simulink model "PONG"  (R2018b)
settings: Solver=VariableStepAuto  StartTime=0.0  StopTime=10  RelTol=1e-3
libraries: simulink_extras x28
(part 2 of 3)

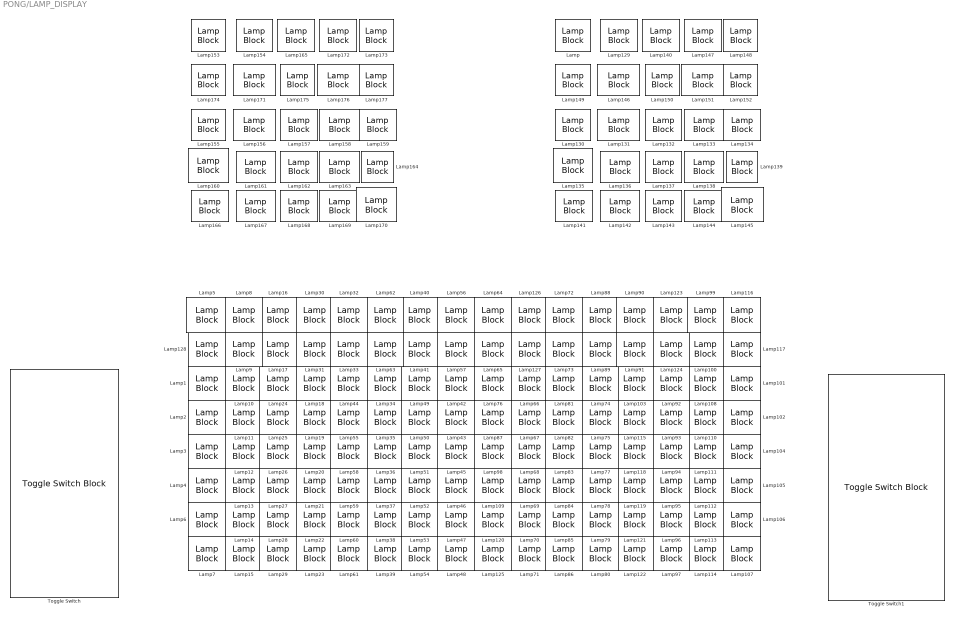
== system PONG/LAMP_DISPLAY  ==
  Lamp : LampBlock  WebBlockId=4723  LabelPosition=Hide
  Lamp1 : LampBlock  WebBlockId=1763  LabelPosition=Hide
  Lamp10 : LampBlock  WebBlockId=1211  LabelPosition=Hide
  Lamp100 : LampBlock  WebBlockId=1301  LabelPosition=Hide
  Lamp101 : LampBlock  WebBlockId=1302  LabelPosition=Hide
  Lamp102 : LampBlock  WebBlockId=1303  LabelPosition=Hide
  Lamp103 : LampBlock  WebBlockId=1304  LabelPosition=Hide
  Lamp104 : LampBlock  WebBlockId=1305  LabelPosition=Hide
  Lamp105 : LampBlock  WebBlockId=1306  LabelPosition=Hide
  Lamp106 : LampBlock  WebBlockId=1307  LabelPosition=Hide
  Lamp107 : LampBlock  WebBlockId=1308  LabelPosition=Hide
  Lamp108 : LampBlock  WebBlockId=1309  LabelPosition=Hide
  Lamp109 : LampBlock  WebBlockId=1310  LabelPosition=Hide
  Lamp11 : LampBlock  WebBlockId=1212  LabelPosition=Hide
  Lamp110 : LampBlock  WebBlockId=1311  LabelPosition=Hide
  Lamp111 : LampBlock  WebBlockId=1312  LabelPosition=Hide
  Lamp112 : LampBlock  WebBlockId=1313  LabelPosition=Hide
  Lamp113 : LampBlock  WebBlockId=1314  LabelPosition=Hide
  Lamp114 : LampBlock  WebBlockId=1315  LabelPosition=Hide
  Lamp115 : LampBlock  WebBlockId=1316  LabelPosition=Hide
  Lamp116 : LampBlock  WebBlockId=1317  LabelPosition=Hide
  Lamp117 : LampBlock  WebBlockId=1318  LabelPosition=Hide
  Lamp118 : LampBlock  WebBlockId=1319  LabelPosition=Hide
  Lamp119 : LampBlock  WebBlockId=1320  LabelPosition=Hide
  Lamp12 : LampBlock  WebBlockId=1213  LabelPosition=Hide
  Lamp120 : LampBlock  WebBlockId=1321  LabelPosition=Hide
  Lamp121 : LampBlock  WebBlockId=1322  LabelPosition=Hide
  Lamp122 : LampBlock  WebBlockId=1323  LabelPosition=Hide
  Lamp123 : LampBlock  WebBlockId=1324  LabelPosition=Hide
  Lamp124 : LampBlock  WebBlockId=1325  LabelPosition=Hide
  Lamp125 : LampBlock  WebBlockId=1326  LabelPosition=Hide
  Lamp126 : LampBlock  WebBlockId=1327  LabelPosition=Hide
  Lamp127 : LampBlock  WebBlockId=1328  LabelPosition=Hide
  Lamp128 : LampBlock  WebBlockId=1768  LabelPosition=Hide
  Lamp129 : LampBlock  WebBlockId=4724  LabelPosition=Hide
  Lamp13 : LampBlock  WebBlockId=1214  LabelPosition=Hide
  Lamp130 : LampBlock  WebBlockId=4725  LabelPosition=Hide
  Lamp131 : LampBlock  WebBlockId=4726  LabelPosition=Hide
  Lamp132 : LampBlock  WebBlockId=4727  LabelPosition=Hide
  Lamp133 : LampBlock  WebBlockId=4728  LabelPosition=Hide
  Lamp134 : LampBlock  WebBlockId=4729  LabelPosition=Hide
  Lamp135 : LampBlock  WebBlockId=4730  LabelPosition=Hide
  Lamp136 : LampBlock  WebBlockId=4731  LabelPosition=Hide
  Lamp137 : LampBlock  WebBlockId=4732  LabelPosition=Hide
  Lamp138 : LampBlock  WebBlockId=4733  LabelPosition=Hide
  Lamp139 : LampBlock  WebBlockId=4734  LabelPosition=Hide
  Lamp14 : LampBlock  WebBlockId=1215  LabelPosition=Hide
  Lamp140 : LampBlock  WebBlockId=4735  LabelPosition=Hide
  Lamp141 : LampBlock  WebBlockId=4736  LabelPosition=Hide
  Lamp142 : LampBlock  WebBlockId=4737  LabelPosition=Hide
  Lamp143 : LampBlock  WebBlockId=4738  LabelPosition=Hide
  Lamp144 : LampBlock  WebBlockId=4739  LabelPosition=Hide
  Lamp145 : LampBlock  WebBlockId=4740  LabelPosition=Hide
  Lamp146 : LampBlock  WebBlockId=4741  LabelPosition=Hide
  Lamp147 : LampBlock  WebBlockId=4742  LabelPosition=Hide
  Lamp148 : LampBlock  WebBlockId=4743  LabelPosition=Hide
  Lamp149 : LampBlock  WebBlockId=4744  LabelPosition=Hide
  Lamp15 : LampBlock  WebBlockId=1216  LabelPosition=Hide
  Lamp150 : LampBlock  WebBlockId=4745  LabelPosition=Hide
  Lamp151 : LampBlock  WebBlockId=4746  LabelPosition=Hide
  Lamp152 : LampBlock  WebBlockId=4747  LabelPosition=Hide
  Lamp153 : LampBlock  WebBlockId=4748  LabelPosition=Hide
  Lamp154 : LampBlock  WebBlockId=4749  LabelPosition=Hide
  Lamp155 : LampBlock  WebBlockId=4750  LabelPosition=Hide
  Lamp156 : LampBlock  WebBlockId=4751  LabelPosition=Hide
  Lamp157 : LampBlock  WebBlockId=4752  LabelPosition=Hide
  Lamp158 : LampBlock  WebBlockId=4753  LabelPosition=Hide
  Lamp159 : LampBlock  WebBlockId=4754  LabelPosition=Hide
  Lamp16 : LampBlock  WebBlockId=1217  LabelPosition=Hide
  Lamp160 : LampBlock  WebBlockId=4755  LabelPosition=Hide
  Lamp161 : LampBlock  WebBlockId=4756  LabelPosition=Hide
  Lamp162 : LampBlock  WebBlockId=4757  LabelPosition=Hide
  Lamp163 : LampBlock  WebBlockId=4758  LabelPosition=Hide
  Lamp164 : LampBlock  WebBlockId=4759  LabelPosition=Hide
  Lamp165 : LampBlock  WebBlockId=4760  LabelPosition=Hide
  Lamp166 : LampBlock  WebBlockId=4761  LabelPosition=Hide
  Lamp167 : LampBlock  WebBlockId=4762  LabelPosition=Hide
  Lamp168 : LampBlock  WebBlockId=4763  LabelPosition=Hide
  Lamp169 : LampBlock  WebBlockId=4764  LabelPosition=Hide
  Lamp17 : LampBlock  WebBlockId=1218  LabelPosition=Hide
  Lamp170 : LampBlock  WebBlockId=4765  LabelPosition=Hide
  Lamp171 : LampBlock  WebBlockId=4766  LabelPosition=Hide
  Lamp172 : LampBlock  WebBlockId=4767  LabelPosition=Hide
  Lamp173 : LampBlock  WebBlockId=4768  LabelPosition=Hide
  Lamp174 : LampBlock  WebBlockId=4769  LabelPosition=Hide
  Lamp175 : LampBlock  WebBlockId=4770  LabelPosition=Hide
  Lamp176 : LampBlock  WebBlockId=4771  LabelPosition=Hide
  Lamp177 : LampBlock  WebBlockId=4772  LabelPosition=Hide
  Lamp18 : LampBlock  WebBlockId=1219  LabelPosition=Hide
  Lamp19 : LampBlock  WebBlockId=1220  LabelPosition=Hide
  Lamp2 : LampBlock  WebBlockId=1764  LabelPosition=Hide
  Lamp20 : LampBlock  WebBlockId=1221  LabelPosition=Hide
  Lamp21 : LampBlock  WebBlockId=1222  LabelPosition=Hide
  Lamp22 : LampBlock  WebBlockId=1223  LabelPosition=Hide
  Lamp23 : LampBlock  WebBlockId=1224  LabelPosition=Hide
  Lamp24 : LampBlock  WebBlockId=1225  LabelPosition=Hide
  Lamp25 : LampBlock  WebBlockId=1226  LabelPosition=Hide
  Lamp26 : LampBlock  WebBlockId=1227  LabelPosition=Hide
  Lamp27 : LampBlock  WebBlockId=1228  LabelPosition=Hide
  Lamp28 : LampBlock  WebBlockId=1229  LabelPosition=Hide
  Lamp29 : LampBlock  WebBlockId=1230  LabelPosition=Hide
  Lamp3 : LampBlock  WebBlockId=1765  LabelPosition=Hide
  Lamp30 : LampBlock  WebBlockId=1231  LabelPosition=Hide
  Lamp31 : LampBlock  WebBlockId=1232  LabelPosition=Hide
  Lamp32 : LampBlock  WebBlockId=1233  LabelPosition=Hide
  Lamp33 : LampBlock  WebBlockId=1234  LabelPosition=Hide
  Lamp34 : LampBlock  WebBlockId=1235  LabelPosition=Hide
  Lamp35 : LampBlock  WebBlockId=1236  LabelPosition=Hide
  Lamp36 : LampBlock  WebBlockId=1237  LabelPosition=Hide
  Lamp37 : LampBlock  WebBlockId=1238  LabelPosition=Hide
  Lamp38 : LampBlock  WebBlockId=1239  LabelPosition=Hide
  Lamp39 : LampBlock  WebBlockId=1240  LabelPosition=Hide
  Lamp4 : LampBlock  WebBlockId=1766  LabelPosition=Hide
  Lamp40 : LampBlock  WebBlockId=1241  LabelPosition=Hide
  Lamp41 : LampBlock  WebBlockId=1242  LabelPosition=Hide
  Lamp42 : LampBlock  WebBlockId=1243  LabelPosition=Hide
  Lamp43 : LampBlock  WebBlockId=1244  LabelPosition=Hide
  Lamp44 : LampBlock  WebBlockId=1245  LabelPosition=Hide
  Lamp45 : LampBlock  WebBlockId=1246  LabelPosition=Hide
  Lamp46 : LampBlock  WebBlockId=1247  LabelPosition=Hide
  Lamp47 : LampBlock  WebBlockId=1248  LabelPosition=Hide
  Lamp48 : LampBlock  WebBlockId=1249  LabelPosition=Hide
  Lamp49 : LampBlock  WebBlockId=1250  LabelPosition=Hide
  Lamp5 : LampBlock  WebBlockId=1767  LabelPosition=Hide
  Lamp50 : LampBlock  WebBlockId=1251  LabelPosition=Hide
  Lamp51 : LampBlock  WebBlockId=1252  LabelPosition=Hide
  Lamp52 : LampBlock  WebBlockId=1253  LabelPosition=Hide
  Lamp53 : LampBlock  WebBlockId=1254  LabelPosition=Hide
  Lamp54 : LampBlock  WebBlockId=1255  LabelPosition=Hide
  Lamp55 : LampBlock  WebBlockId=1256  LabelPosition=Hide
  Lamp56 : LampBlock  WebBlockId=1257  LabelPosition=Hide
  Lamp57 : LampBlock  WebBlockId=1258  LabelPosition=Hide
  Lamp58 : LampBlock  WebBlockId=1259  LabelPosition=Hide
  Lamp59 : LampBlock  WebBlockId=1260  LabelPosition=Hide
  Lamp6 : LampBlock  WebBlockId=1207  LabelPosition=Hide
  Lamp60 : LampBlock  WebBlockId=1261  LabelPosition=Hide
  Lamp61 : LampBlock  WebBlockId=1262  LabelPosition=Hide
  Lamp62 : LampBlock  WebBlockId=1263  LabelPosition=Hide
  Lamp63 : LampBlock  WebBlockId=1264  LabelPosition=Hide
  Lamp64 : LampBlock  WebBlockId=1265  LabelPosition=Hide
  Lamp65 : LampBlock  WebBlockId=1266  LabelPosition=Hide
  Lamp66 : LampBlock  WebBlockId=1267  LabelPosition=Hide
  Lamp67 : LampBlock  WebBlockId=1268  LabelPosition=Hide
  Lamp68 : LampBlock  WebBlockId=1269  LabelPosition=Hide
  Lamp69 : LampBlock  WebBlockId=1270  LabelPosition=Hide
  Lamp7 : LampBlock  WebBlockId=1208  LabelPosition=Hide
  Lamp70 : LampBlock  WebBlockId=1271  LabelPosition=Hide
  Lamp71 : LampBlock  WebBlockId=1272  LabelPosition=Hide
  Lamp72 : LampBlock  WebBlockId=1273  LabelPosition=Hide
  Lamp73 : LampBlock  WebBlockId=1274  LabelPosition=Hide
  Lamp74 : LampBlock  WebBlockId=1275  LabelPosition=Hide
  Lamp75 : LampBlock  WebBlockId=1276  LabelPosition=Hide
  Lamp76 : LampBlock  WebBlockId=1277  LabelPosition=Hide
  Lamp77 : LampBlock  WebBlockId=1278  LabelPosition=Hide
  Lamp78 : LampBlock  WebBlockId=1279  LabelPosition=Hide
  Lamp79 : LampBlock  WebBlockId=1280  LabelPosition=Hide
  Lamp8 : LampBlock  WebBlockId=1209  LabelPosition=Hide
  Lamp80 : LampBlock  WebBlockId=1281  LabelPosition=Hide
  Lamp81 : LampBlock  WebBlockId=1282  LabelPosition=Hide
  Lamp82 : LampBlock  WebBlockId=1283  LabelPosition=Hide
  Lamp83 : LampBlock  WebBlockId=1284  LabelPosition=Hide
  Lamp84 : LampBlock  WebBlockId=1285  LabelPosition=Hide
  Lamp85 : LampBlock  WebBlockId=1286  LabelPosition=Hide
  Lamp86 : LampBlock  WebBlockId=1287  LabelPosition=Hide
  Lamp87 : LampBlock  WebBlockId=1288  LabelPosition=Hide
  Lamp88 : LampBlock  WebBlockId=1289  LabelPosition=Hide
  Lamp89 : LampBlock  WebBlockId=1290  LabelPosition=Hide
  Lamp9 : LampBlock  WebBlockId=1210  LabelPosition=Hide
  Lamp90 : LampBlock  WebBlockId=1291  LabelPosition=Hide
  Lamp91 : LampBlock  WebBlockId=1292  LabelPosition=Hide
  Lamp92 : LampBlock  WebBlockId=1293  LabelPosition=Hide
  Lamp93 : LampBlock  WebBlockId=1294  LabelPosition=Hide
  Lamp94 : LampBlock  WebBlockId=1295  LabelPosition=Hide
  Lamp95 : LampBlock  WebBlockId=1296  LabelPosition=Hide
  Lamp96 : LampBlock  WebBlockId=1297  LabelPosition=Hide
  Lamp97 : LampBlock  WebBlockId=1298  LabelPosition=Hide
  Lamp98 : LampBlock  WebBlockId=1299  LabelPosition=Hide
  Lamp99 : LampBlock  WebBlockId=1300  LabelPosition=Hide
  Toggle Switch : ToggleSwitchBlock  WebBlockId=3885  LabelPosition=Hide
      settings: Values={{'Down', 'Up'}, [1 0]}
  Toggle Switch1 : ToggleSwitchBlock  WebBlockId=3886  LabelPosition=Hide
      settings: Values={{'Down', 'Up'}, [1 0]}

== system PONG/Next State  ==
  CLK 1 : Inport
  EN_Xball1 : Inport  Port=2
  EN_Yball1 : Inport  Port=3
  EN_Yball0 : Inport  Port=4
  "EN_reset " : Inport  Port=5
  MOVE_XBall_CONTROLLED ( EN=0 >Right ;  EN=1 > left ) 3 : Subsystem  TreatAsAtomicUnit=on
  MOVE_YBall_CONTROLLED ( EN=0 >Up ;  EN=1 > Down ) 3 : Subsystem  TreatAsAtomicUnit=on
  Scope : Scope  NumInputPorts=7
  A1 : Outport
  B1 : Outport  Port=2
  C1 : Outport  Port=3
  D1 : Outport  Port=4
  E1 : Outport  Port=5
  F1 : Outport  Port=6
  G1 : Outport  Port=7
  wires:
  CLK 1/1 -> MOVE_YBall_CONTROLLED ( EN=0 >Up ;  EN=1 > Down ) 3/1(CLK), MOVE_XBall_CONTROLLED ( EN=0 >Right ;  EN=1 > left ) 3/1("CLK ")
  MOVE_XBall_CONTROLLED ( EN=0 >Right ;  EN=1 > left ) 3/4(D) -> Scope/4, D1/1
  MOVE_XBall_CONTROLLED ( EN=0 >Right ;  EN=1 > left ) 3/2(B) -> Scope/2, B1/1
  MOVE_XBall_CONTROLLED ( EN=0 >Right ;  EN=1 > left ) 3/1(A) -> Scope/1, A1/1
  MOVE_YBall_CONTROLLED ( EN=0 >Up ;  EN=1 > Down ) 3/3(G) -> Scope/7, G1/1
  MOVE_YBall_CONTROLLED ( EN=0 >Up ;  EN=1 > Down ) 3/1(E) -> Scope/5, E1/1
  MOVE_YBall_CONTROLLED ( EN=0 >Up ;  EN=1 > Down ) 3/2(F) -> Scope/6, F1/1
  "EN_reset "/1 -> MOVE_XBall_CONTROLLED ( EN=0 >Right ;  EN=1 > left ) 3/3(EN_reset), MOVE_YBall_CONTROLLED ( EN=0 >Up ;  EN=1 > Down ) 3/4(EN_reset)
  MOVE_XBall_CONTROLLED ( EN=0 >Right ;  EN=1 > left ) 3/3(C) -> Scope/3, C1/1
  EN_Xball1/1 -> MOVE_XBall_CONTROLLED ( EN=0 >Right ;  EN=1 > left ) 3/2("EN ")
  EN_Yball1/1 -> MOVE_YBall_CONTROLLED ( EN=0 >Up ;  EN=1 > Down ) 3/2(EN1)
  EN_Yball0/1 -> MOVE_YBall_CONTROLLED ( EN=0 >Up ;  EN=1 > Down ) 3/3(EN0)

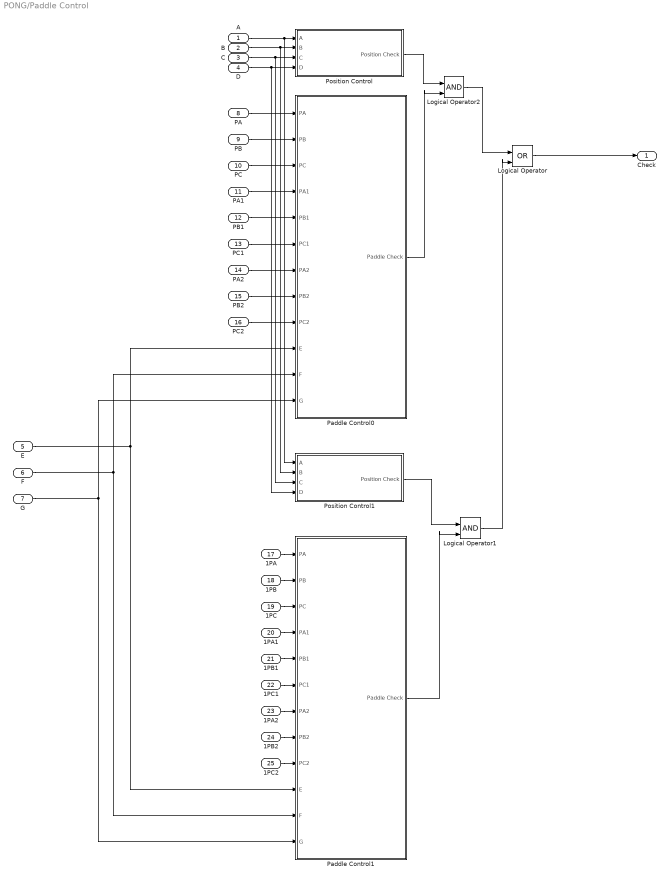
== system PONG/Paddle Control ==
  A : Inport
  B : Inport  Port=2
  C : Inport  Port=3
  D : Inport  Port=4
  E : Inport  Port=5
  F : Inport  Port=6
  G : Inport  Port=7
  PA : Inport  Port=8
  PB : Inport  Port=9
  PC : Inport  Port=10
  PA1 : Inport  Port=11
  PB1 : Inport  Port=12
  PC1 : Inport  Port=13
  PA2 : Inport  Port=14
  PB2 : Inport  Port=15
  PC2 : Inport  Port=16
  1PA : Inport  Port=17
  1PB : Inport  Port=18
  1PC : Inport  Port=19
  1PA1 : Inport  Port=20
  1PB1 : Inport  Port=21
  1PC1 : Inport  Port=22
  1PA2 : Inport  Port=23
  1PB2 : Inport  Port=24
  1PC2 : Inport  Port=25
  Logical Operator : Logic  Operator=OR  IconShape=distinctive  AllPortsSameDT=off  OutDataTypeStr=boolean
  Logical Operator1 : Logic  IconShape=distinctive  AllPortsSameDT=off  OutDataTypeStr=boolean
  Logical Operator2 : Logic  IconShape=distinctive  AllPortsSameDT=off  OutDataTypeStr=boolean
  Paddle Control0 : Subsystem  TreatAsAtomicUnit=on
  Paddle Control1 : Subsystem  TreatAsAtomicUnit=on
  Position Control : Subsystem  TreatAsAtomicUnit=on
  Position Control1 : Subsystem  TreatAsAtomicUnit=on
  Check : Outport
  wires:
  B/1 -> Position Control1/2(B), Position Control/2(B)
  C/1 -> Position Control1/3(C), Position Control/3(C)
  D/1 -> Position Control1/4(D), Position Control/4(D)
  F/1 -> Paddle Control1/11(F), Paddle Control0/11(F)
  PC2/1 -> Paddle Control0/9(PC2)
  PB2/1 -> Paddle Control0/8(PB2)
  PA2/1 -> Paddle Control0/7(PA2)
  PC1/1 -> Paddle Control0/6(PC1)
  PB1/1 -> Paddle Control0/5(PB1)
  PA1/1 -> Paddle Control0/4(PA1)
  PC/1 -> Paddle Control0/3(PC)
  PA/1 -> Paddle Control0/1(PA)
  PB/1 -> Paddle Control0/2(PB)
  E/1 -> Paddle Control1/10(E), Paddle Control0/10(E)
  G/1 -> Paddle Control1/12(G), Paddle Control0/12(G)
  1PC2/1 -> Paddle Control1/9(PC2)
  1PB2/1 -> Paddle Control1/8(PB2)
  1PA2/1 -> Paddle Control1/7(PA2)
  1PC1/1 -> Paddle Control1/6(PC1)
  1PB1/1 -> Paddle Control1/5(PB1)
  1PA1/1 -> Paddle Control1/4(PA1)
  1PC/1 -> Paddle Control1/3(PC)
  1PB/1 -> Paddle Control1/2(PB)
  1PA/1 -> Paddle Control1/1(PA)
  Logical Operator/1 -> Check/1
  Paddle Control1/1(Paddle Check) -> Logical Operator1/2
  Logical Operator1/1 -> Logical Operator/2
  Logical Operator2/1 -> Logical Operator/1
  Position Control/1(Position Check) -> Logical Operator2/1
  A/1 -> Position Control1/1(A), Position Control/1(A)
  Paddle Control0/1(Paddle Check) -> Logical Operator2/2
  Position Control1/1(Position Check) -> Logical Operator1/1

== system PONG/Paddle DEMUXER0 ==
  PA0 : Inport
  PB0 : Inport  Port=2
  PC0 : Inport  Port=3
  PA1 : Inport  Port=4
  PB1 : Inport  Port=5
  PC1 : Inport  Port=6
  PA2 : Inport  Port=7
  PB2 : Inport  Port=8
  PC2 : Inport  Port=9
  1PaddleDEMUXER0 : Subsystem
  1PaddleDEMUXER2 : Subsystem
  2PaddleDEMUXER1 : Subsystem
  Logical Operator{,1..7} (8 alike) : Logic  Operator=OR  Inputs=3  IconShape=distinctive  AllPortsSameDT=off  OutDataTypeStr=boolean
  000 : Outport
  001 : Outport  Port=2
  010 : Outport  Port=3
  011 : Outport  Port=4
  100 : Outport  Port=5
  101 : Outport  Port=6
  110 : Outport  Port=7
  111 : Outport  Port=8
  wires:
  Logical Operator/1 -> 000/1
  Logical Operator1/1 -> 001/1
  Logical Operator3/1 -> 011/1
  Logical Operator2/1 -> 010/1
  Logical Operator6/1 -> 110/1
  Logical Operator7/1 -> 111/1
  Logical Operator5/1 -> 101/1
  Logical Operator4/1 -> 100/1
  2PaddleDEMUXER1/1(Out1) -> Logical Operator/2
  1PaddleDEMUXER0/1(Out1) -> Logical Operator/1
  1PaddleDEMUXER2/1(Out1) -> Logical Operator/3
  1PaddleDEMUXER0/2(Out2) -> Logical Operator1/1
  2PaddleDEMUXER1/2(Out2) -> Logical Operator1/2
  1PaddleDEMUXER2/2(Out2) -> Logical Operator1/3
  1PaddleDEMUXER0/3(Out3) -> Logical Operator2/1
  2PaddleDEMUXER1/3(Out3) -> Logical Operator2/2
  1PaddleDEMUXER2/3(Out3) -> Logical Operator2/3
  1PaddleDEMUXER0/4(Out4) -> Logical Operator3/1
  2PaddleDEMUXER1/4(Out4) -> Logical Operator3/2
  1PaddleDEMUXER2/4(Out4) -> Logical Operator3/3
  1PaddleDEMUXER0/5(Out5) -> Logical Operator4/1
  2PaddleDEMUXER1/5(Out5) -> Logical Operator4/2
  1PaddleDEMUXER2/5(Out5) -> Logical Operator4/3
  2PaddleDEMUXER1/6(Out6) -> Logical Operator5/2
  1PaddleDEMUXER0/6(Out6) -> Logical Operator5/1
  1PaddleDEMUXER2/6(Out6) -> Logical Operator5/3
  1PaddleDEMUXER0/7(Out7) -> Logical Operator6/1
  2PaddleDEMUXER1/7(Out7) -> Logical Operator6/2
  1PaddleDEMUXER2/7(Out7) -> Logical Operator6/3
  1PaddleDEMUXER2/8(Out8) -> Logical Operator7/3
  2PaddleDEMUXER1/8(Out8) -> Logical Operator7/2
  1PaddleDEMUXER0/8(Out8) -> Logical Operator7/1
  PA0/1 -> 1PaddleDEMUXER0/3(PC)
  PB0/1 -> 1PaddleDEMUXER0/2(PB)
  PC0/1 -> 1PaddleDEMUXER0/1(PA)
  PC2/1 -> 1PaddleDEMUXER2/3(PC)
  PA1/1 -> 2PaddleDEMUXER1/1(PA)
  PB1/1 -> 2PaddleDEMUXER1/2(PB)
  PC1/1 -> 2PaddleDEMUXER1/3(PC)
  PA2/1 -> 1PaddleDEMUXER2/1(PA)
  PB2/1 -> 1PaddleDEMUXER2/2(PB)

== system PONG/Paddle DEMUXER1 ==
  PA0 : Inport
  PB0 : Inport  Port=2
  PC0 : Inport  Port=3
  PA1 : Inport  Port=4
  PB1 : Inport  Port=5
  PC1 : Inport  Port=6
  PA2 : Inport  Port=7
  PB2 : Inport  Port=8
  PC2 : Inport  Port=9
  1PaddleDEMUXER0 : Subsystem
  1PaddleDEMUXER1 : Subsystem
  1PaddleDEMUXER2 : Subsystem
  Logical Operator{,1..7} (8 alike) : Logic  Operator=OR  Inputs=3  IconShape=distinctive  AllPortsSameDT=off  OutDataTypeStr=boolean
  000 : Outport
  001 : Outport  Port=2
  010 : Outport  Port=3
  011 : Outport  Port=4
  100 : Outport  Port=5
  101 : Outport  Port=6
  110 : Outport  Port=7
  111 : Outport  Port=8
  wires:
  PB2/1 -> 1PaddleDEMUXER2/2(PB)
  PA2/1 -> 1PaddleDEMUXER2/1(PA)
  PC1/1 -> 1PaddleDEMUXER1/3(PC)
  PB1/1 -> 1PaddleDEMUXER1/2(PB)
  PA1/1 -> 1PaddleDEMUXER1/1(PA)
  PC2/1 -> 1PaddleDEMUXER2/3(PC)
  PC0/1 -> 1PaddleDEMUXER0/3(PC)
  PB0/1 -> 1PaddleDEMUXER0/2(PB)
  PA0/1 -> 1PaddleDEMUXER0/1(PA)
  1PaddleDEMUXER0/8(Out8) -> Logical Operator7/1
  1PaddleDEMUXER1/8(Out8) -> Logical Operator7/2
  1PaddleDEMUXER2/8(Out8) -> Logical Operator7/3
  1PaddleDEMUXER2/7(Out7) -> Logical Operator6/3
  1PaddleDEMUXER1/7(Out7) -> Logical Operator6/2
  1PaddleDEMUXER0/7(Out7) -> Logical Operator6/1
  1PaddleDEMUXER2/6(Out6) -> Logical Operator5/3
  1PaddleDEMUXER0/6(Out6) -> Logical Operator5/1
  1PaddleDEMUXER1/6(Out6) -> Logical Operator5/2
  1PaddleDEMUXER2/5(Out5) -> Logical Operator4/3
  1PaddleDEMUXER1/5(Out5) -> Logical Operator4/2
  1PaddleDEMUXER0/5(Out5) -> Logical Operator4/1
  1PaddleDEMUXER2/4(Out4) -> Logical Operator3/3
  1PaddleDEMUXER1/4(Out4) -> Logical Operator3/2
  1PaddleDEMUXER0/4(Out4) -> Logical Operator3/1
  1PaddleDEMUXER2/3(Out3) -> Logical Operator2/3
  1PaddleDEMUXER1/3(Out3) -> Logical Operator2/2
  1PaddleDEMUXER0/3(Out3) -> Logical Operator2/1
  1PaddleDEMUXER2/2(Out2) -> Logical Operator1/3
  1PaddleDEMUXER1/2(Out2) -> Logical Operator1/2
  1PaddleDEMUXER0/2(Out2) -> Logical Operator1/1
  1PaddleDEMUXER2/1(Out1) -> Logical Operator/3
  1PaddleDEMUXER0/1(Out1) -> Logical Operator/1
  1PaddleDEMUXER1/1(Out1) -> Logical Operator/2
  Logical Operator4/1 -> 100/1
  Logical Operator5/1 -> 101/1
  Logical Operator7/1 -> 111/1
  Logical Operator6/1 -> 110/1
  Logical Operator2/1 -> 010/1
  Logical Operator3/1 -> 011/1
  Logical Operator1/1 -> 001/1
  Logical Operator/1 -> 000/1

== system PONG/Paddle0 ==
  Controller : Inport
  CLK : Inport  Port=2
  Atomic Subsystem : Subsystem  TreatAsAtomicUnit=on
  Atomic Subsystem1 : Subsystem  TreatAsAtomicUnit=on
  Atomic Subsystem2 : Subsystem  TreatAsAtomicUnit=on
  Atomic Subsystem3 : Subsystem  TreatAsAtomicUnit=on
  Mux : Mux  Inputs=3
  Mux1 : Mux  Inputs=3
  Mux2 : Mux  Inputs=3
  Scope : Scope
  Scope1 : Scope
  Scope2 : Scope
  PA : Outport
  PB : Outport  Port=2
  PC : Outport  Port=3
  PA1 : Outport  Port=4
  PB1 : Outport  Port=5
  PC1 : Outport  Port=6
  PA2 : Outport  Port=7
  PB2 : Outport  Port=8
  PC2 : Outport  Port=9
  wires:
  Atomic Subsystem3/2(PB0) -> Atomic Subsystem2/2(PB0), Atomic Subsystem1/2(PB0), Mux/2, PB/1
  Atomic Subsystem3/3(PC0) -> Atomic Subsystem2/3(PC0), Atomic Subsystem1/3(PC0), Mux/3, PC/1
  Atomic Subsystem3/1(PA0) -> Atomic Subsystem2/1(PA0), Atomic Subsystem1/1(PA0), Mux/1, PA/1
  Mux/1 -> Scope/1
  Mux1/1 -> Scope1/1
  Atomic Subsystem1/1(PA1) -> Mux1/1, PA1/1
  Atomic Subsystem1/3(PC1) -> Mux1/3, PC1/1
  Atomic Subsystem1/2(PB1) -> Mux1/2, PB1/1
  Atomic Subsystem2/2(PB1) -> Mux2/2, PB2/1
  Atomic Subsystem2/3(PC1) -> Mux2/3, PC2/1
  Atomic Subsystem2/1(PA1) -> Mux2/1, PA2/1
  Mux2/1 -> Scope2/1
  CLK/1 -> Atomic Subsystem3/1(CLK)
  Controller/1 -> Atomic Subsystem3/2(Ctrl)

== system PONG/Paddle1 ==
  Controller : Inport
  CLK : Inport  Port=2
  Atomic Subsystem1 : Subsystem  TreatAsAtomicUnit=on
  Atomic Subsystem2 : Subsystem  TreatAsAtomicUnit=on
  Atomic Subsystem3 : Subsystem  TreatAsAtomicUnit=on
  Mux : Mux  Inputs=3
  Mux1 : Mux  Inputs=3
  Mux2 : Mux  Inputs=3
  Scope : Scope
  Scope1 : Scope
  Scope2 : Scope
  PA : Outport
  PB : Outport  Port=2
  PC : Outport  Port=3
  PA1 : Outport  Port=4
  PB1 : Outport  Port=5
  PC1 : Outport  Port=6
  PA2 : Outport  Port=7
  PB2 : Outport  Port=8
  PC2 : Outport  Port=9
  wires:
  Controller/1 -> Atomic Subsystem3/2(Ctrl)
  CLK/1 -> Atomic Subsystem3/1(CLK)
  Mux2/1 -> Scope2/1
  Atomic Subsystem2/1(PA1) -> PA2/1, Mux2/1
  Atomic Subsystem2/3(PC1) -> PC2/1, Mux2/3
  Atomic Subsystem2/2(PB1) -> PB2/1, Mux2/2
  Atomic Subsystem1/2(PB1) -> PB1/1, Mux1/2
  Atomic Subsystem1/3(PC1) -> PC1/1, Mux1/3
  Atomic Subsystem1/1(PA1) -> PA1/1, Mux1/1
  Mux1/1 -> Scope1/1
  Mux/1 -> Scope/1
  Atomic Subsystem3/1(PA0) -> PA/1, Mux/1, Atomic Subsystem1/1(PA0), Atomic Subsystem2/1(PA0)
  Atomic Subsystem3/3(PC0) -> PC/1, Mux/3, Atomic Subsystem1/3(PC0), Atomic Subsystem2/3(PC0)
  Atomic Subsystem3/2(PB0) -> PB/1, Mux/2, Atomic Subsystem1/2(PB0), Atomic Subsystem2/2(PB0)

== system PONG/PointReset ==
  A : Inport
  B : Inport  Port=2
  C : Inport  Port=3
  D : Inport  Port=4
  Logical Operator : Logic  Operator=NXOR  IconShape=distinctive  AllPortsSameDT=off  OutDataTypeStr=boolean
  Logical Operator1 : Logic  Operator=NXOR  IconShape=distinctive  AllPortsSameDT=off  OutDataTypeStr=boolean
  Logical Operator2 : Logic  Operator=NXOR  IconShape=distinctive  AllPortsSameDT=off  OutDataTypeStr=boolean
  Logical Operator3 : Logic  Inputs=3  IconShape=distinctive  AllPortsSameDT=off  OutDataTypeStr=boolean
  PointReset : Outport
  Winner : Outport  Port=2
  wires:
  A/1 -> Logical Operator/1
  B/1 -> Logical Operator2/1, Logical Operator/2
  C/1 -> Logical Operator1/1, Logical Operator2/2
  D/1 -> Winner/1, Logical Operator1/2
  Logical Operator2/1 -> Logical Operator3/2
  Logical Operator3/1 -> PointReset/1
  Logical Operator/1 -> Logical Operator3/1
  Logical Operator1/1 -> Logical Operator3/3

== system PONG/Subsystem ==
  En : Inport
  CLK : Inport  Port=2
  Combinational Logic for the matrix of leds-from 0 to 9 (No2) : Subsystem
  Counter from 0 to 9 : Subsystem
  wires:
  Combinational Logic for the matrix of leds-from 0 to 9 (No2)/17(t1) -> ?
  Combinational Logic for the matrix of leds-from 0 to 9 (No2)/10(l1) -> ?
  Combinational Logic for the matrix of leds-from 0 to 9 (No2)/13(ñ1) -> ?
  Combinational Logic for the matrix of leds-from 0 to 9 (No2)/5(e1) -> ?
  Combinational Logic for the matrix of leds-from 0 to 9 (No2)/8(j1) -> ?
  Combinational Logic for the matrix of leds-from 0 to 9 (No2)/2(b1) -> ?
  Counter from 0 to 9/1(A) -> Combinational Logic for the matrix of leds-from 0 to 9 (No2)/1(A)
  Combinational Logic for the matrix of leds-from 0 to 9 (No2)/7(h1) -> ?
  Combinational Logic for the matrix of leds-from 0 to 9 (No2)/3(c1) -> ?
  Combinational Logic for the matrix of leds-from 0 to 9 (No2)/15(q1) -> ?
  Combinational Logic for the matrix of leds-from 0 to 9 (No2)/14(o1) -> ?
  Combinational Logic for the matrix of leds-from 0 to 9 (No2)/9(k1) -> ?
  Combinational Logic for the matrix of leds-from 0 to 9 (No2)/20(w1) -> ?
  Combinational Logic for the matrix of leds-from 0 to 9 (No2)/1(a1) -> ?
  Combinational Logic for the matrix of leds-from 0 to 9 (No2)/18(u1) -> ?
  Combinational Logic for the matrix of leds-from 0 to 9 (No2)/19(v1) -> ?
  Combinational Logic for the matrix of leds-from 0 to 9 (No2)/11(m1) -> ?
  Counter from 0 to 9/3(C) -> Combinational Logic for the matrix of leds-from 0 to 9 (No2)/3(C)
  Combinational Logic for the matrix of leds-from 0 to 9 (No2)/6(f1) -> ?
  Combinational Logic for the matrix of leds-from 0 to 9 (No2)/21(x1) -> ?
  Combinational Logic for the matrix of leds-from 0 to 9 (No2)/4(d1) -> ?
  Combinational Logic for the matrix of leds-from 0 to 9 (No2)/16(s1) -> ?
  Combinational Logic for the matrix of leds-from 0 to 9 (No2)/22(zero1) -> ?
  Combinational Logic for the matrix of leds-from 0 to 9 (No2)/12(n1) -> ?
  Counter from 0 to 9/2(B) -> Combinational Logic for the matrix of leds-from 0 to 9 (No2)/2(B)
  Counter from 0 to 9/4(D) -> Combinational Logic for the matrix of leds-from 0 to 9 (No2)/4(D)
  En/1 -> Counter from 0 to 9/1(EN)
  CLK/1 -> Counter from 0 to 9/2(CLK)

== system PONG/Subsystem2 ==
  EN : Inport
  CLK : Inport  Port=2
  Combinational Logic for the matrix of leds-from 0 to 9 : Subsystem
  Counter from 0 to 9 : Subsystem
  wires:
  Combinational Logic for the matrix of leds-from 0 to 9/20(w) -> ?
  Combinational Logic for the matrix of leds-from 0 to 9/21(x) -> ?
  Combinational Logic for the matrix of leds-from 0 to 9/19(v) -> ?
  Combinational Logic for the matrix of leds-from 0 to 9/17(t) -> ?
  Combinational Logic for the matrix of leds-from 0 to 9/18(u) -> ?
  Combinational Logic for the matrix of leds-from 0 to 9/11(m) -> ?
  Combinational Logic for the matrix of leds-from 0 to 9/12(n) -> ?
  Combinational Logic for the matrix of leds-from 0 to 9/22(zero) -> ?
  Combinational Logic for the matrix of leds-from 0 to 9/13(ñ) -> ?
  Combinational Logic for the matrix of leds-from 0 to 9/14(o) -> ?
  Combinational Logic for the matrix of leds-from 0 to 9/15(q) -> ?
  Combinational Logic for the matrix of leds-from 0 to 9/16(s) -> ?
  Combinational Logic for the matrix of leds-from 0 to 9/7(h) -> ?
  Combinational Logic for the matrix of leds-from 0 to 9/10(l) -> ?
  Combinational Logic for the matrix of leds-from 0 to 9/6(f) -> ?
  Combinational Logic for the matrix of leds-from 0 to 9/9(k) -> ?
  Combinational Logic for the matrix of leds-from 0 to 9/1(a) -> ?
  Combinational Logic for the matrix of leds-from 0 to 9/2(b) -> ?
  Combinational Logic for the matrix of leds-from 0 to 9/8(j) -> ?
  Combinational Logic for the matrix of leds-from 0 to 9/3(c) -> ?
  Combinational Logic for the matrix of leds-from 0 to 9/5(e) -> ?
  Combinational Logic for the matrix of leds-from 0 to 9/4(d) -> ?
  EN/1 -> Counter from 0 to 9/1(EN)
  CLK/1 -> Counter from 0 to 9/2(CLK)
  Counter from 0 to 9/4(D) -> Combinational Logic for the matrix of leds-from 0 to 9/4(D)
  Counter from 0 to 9/3(C) -> Combinational Logic for the matrix of leds-from 0 to 9/3(C)
  Counter from 0 to 9/2(B) -> Combinational Logic for the matrix of leds-from 0 to 9/2(B)
  Counter from 0 to 9/1(A) -> Combinational Logic for the matrix of leds-from 0 to 9/1(A)

== system PONG/Vertical Bounce2 ==
  Winner : Inport
  PointReset : Inport  Port=2
  Logical Operator : Logic  IconShape=distinctive  AllPortsSameDT=off  OutDataTypeStr=boolean
  Logical Operator1 : Logic  IconShape=distinctive  AllPortsSameDT=off  OutDataTypeStr=boolean
  Logical Operator2 : Logic  Operator=NOT  IconShape=distinctive  AllPortsSameDT=off  OutDataTypeStr=boolean
  Point0 : Outport
  Point1 : Outport  Port=2
  wires:
  Logical Operator/1 -> Point0/1
  Logical Operator1/1 -> Point1/1
  PointReset/1 -> Logical Operator1/2, Logical Operator/1
  Winner/1 -> Logical Operator/2, Logical Operator2/1
  Logical Operator2/1 -> Logical Operator1/1

== system PONG/Vertical Bounce3 ==
  Check : Inport
  Ctrl0 : Inport  Port=2
  Ctrl1 : Inport  Port=3
  A : Inport  Port=4
  CLK : Inport  Port=5
  E : Inport  Port=6
  F : Inport  Port=7
  G : Inport  Port=8
  J-K Flip-Flop : simulink_extras/Flip Flops/J-K Flip-Flop  initial_condition=0
      settings: SourceProductName=Simulink
  J-K Flip-Flop1 : simulink_extras/Flip Flops/J-K Flip-Flop  initial_condition=0
      settings: SourceProductName=Simulink
  Logical Operator{1,6,10..11,16} (5 alike) : Logic  IconShape=distinctive  AllPortsSameDT=off  OutDataTypeStr=boolean
  Logical Operator12 : Logic  Operator=OR  IconShape=distinctive  AllPortsSameDT=off  OutDataTypeStr=boolean
  Logical Operator13 : Logic  Operator=NOT  Inputs=3  IconShape=distinctive  AllPortsSameDT=off  OutDataTypeStr=boolean
  Logical Operator15 : Logic  Operator=NXOR  IconShape=distinctive  AllPortsSameDT=off  OutDataTypeStr=boolean
  Logical Operator2 : Logic  Operator=OR  IconShape=distinctive  AllPortsSameDT=off  OutDataTypeStr=boolean
  Logical Operator3 : Logic  Operator=OR  Inputs=3  IconShape=distinctive  AllPortsSameDT=off  OutDataTypeStr=boolean
  Logical Operator4 : Logic  Inputs=3  IconShape=distinctive  AllPortsSameDT=off  OutDataTypeStr=boolean
  Logical Operator5 : Logic  Inputs=4  IconShape=distinctive  AllPortsSameDT=off  OutDataTypeStr=boolean
  Logical Operator7 : Logic  Operator=XOR  IconShape=distinctive  AllPortsSameDT=off  OutDataTypeStr=boolean
  Logical Operator8 : Logic  Operator=NXOR  IconShape=distinctive  AllPortsSameDT=off  OutDataTypeStr=boolean
  Logical Operator9 : Logic  Operator=NOT  Inputs=3  IconShape=distinctive  AllPortsSameDT=off  OutDataTypeStr=boolean
  VEnable 1 : Outport
  VEnable 0 : Outport  Port=2
  wires:
  Check/1 -> Logical Operator5/1, Logical Operator4/1, Logical Operator6/1, Logical Operator1/2
  Ctrl0/1 -> Logical Operator11/2
  Logical Operator9/1 -> Logical Operator4/2, Logical Operator7/1
  Logical Operator2/1 -> J-K Flip-Flop/3, J-K Flip-Flop/1
  J-K Flip-Flop/1 -> VEnable 1/1
  Logical Operator3/1 -> J-K Flip-Flop1/3, J-K Flip-Flop1/1
  J-K Flip-Flop1/1 -> VEnable 0/1, Logical Operator4/3, Logical Operator7/2
  CLK/1 -> J-K Flip-Flop1/2, J-K Flip-Flop/2
  A/1 -> Logical Operator10/2, Logical Operator13/1
  Logical Operator13/1 -> Logical Operator11/1
  Ctrl1/1 -> Logical Operator10/1
  Logical Operator10/1 -> Logical Operator12/1
  Logical Operator11/1 -> Logical Operator12/2
  Logical Operator12/1 -> Logical Operator5/2, Logical Operator9/1
  Logical Operator1/1 -> Logical Operator2/1
  Logical Operator4/1 -> Logical Operator3/1
  Logical Operator5/1 -> Logical Operator3/2
  Logical Operator6/1 -> Logical Operator2/2
  J-K Flip-Flop/2 -> Logical Operator1/1, Logical Operator5/3
  J-K Flip-Flop1/2 -> Logical Operator5/4
  Logical Operator7/1 -> Logical Operator6/2
  Logical Operator8/1 -> Logical Operator16/1
  G/1 -> Logical Operator15/2
  F/1 -> Logical Operator15/1, Logical Operator8/2
  E/1 -> Logical Operator8/1
  Logical Operator15/1 -> Logical Operator16/2
  Logical Operator16/1 -> Logical Operator3/3

== system PONG/Next State /MOVE_XBall_CONTROLLED ( EN=0 >Right ;  EN=1 > left ) 3 ==
  "CLK " : Inport
  "EN " : Inport  Port=2
  EN_reset : Inport  Port=3
  Constant : Constant  OutDataTypeStr=boolean
  J-K Flip-Flop : simulink_extras/Flip Flops/J-K Flip-Flop  initial_condition=1
      settings: SourceProductName=Simulink
  J-K Flip-Flop1 : simulink_extras/Flip Flops/J-K Flip-Flop  initial_condition=1
      settings: SourceProductName=Simulink
  J-K Flip-Flop2 : simulink_extras/Flip Flops/J-K Flip-Flop  initial_condition=1
      settings: SourceProductName=Simulink
  J-K Flip-Flop3 : simulink_extras/Flip Flops/J-K Flip-Flop  initial_condition=0
      settings: SourceProductName=Simulink
  Logical Operator10 : Logic  Operator=OR  IconShape=distinctive  AllPortsSameDT=off  OutDataTypeStr=boolean
  Logical Operator{8..9,11,14..16} (6 alike) : Logic  IconShape=distinctive  AllPortsSameDT=off  OutDataTypeStr=boolean
  Logical Operator12 : Logic  Operator=OR  IconShape=distinctive  AllPortsSameDT=off  OutDataTypeStr=boolean
  Logical Operator13 : Logic  Operator=OR  IconShape=distinctive  AllPortsSameDT=off  OutDataTypeStr=boolean
  NOT2 : Logic  Operator=NOT  IconShape=distinctive  AllPortsSameDT=off  OutDataTypeStr=boolean
  Reset_Control1 : Subsystem  TreatAsAtomicUnit=on
  Reset_Control2 : Subsystem  TreatAsAtomicUnit=on
  Reset_Control3 : Subsystem  TreatAsAtomicUnit=on
  Reset_Control4 : Subsystem  TreatAsAtomicUnit=on
  A : Outport
  B : Outport  Port=2
  C : Outport  Port=3
  D : Outport  Port=4
  wires:
  "CLK "/1 -> J-K Flip-Flop1/2, J-K Flip-Flop2/2, J-K Flip-Flop3/2, J-K Flip-Flop/2
  J-K Flip-Flop2/1 -> Logical Operator11/2, B/1
  J-K Flip-Flop1/1 -> C/1, Logical Operator14/2
  J-K Flip-Flop/1 -> D/1, Logical Operator8/2
  J-K Flip-Flop3/1 -> A/1
  J-K Flip-Flop/2 -> Logical Operator9/1
  Logical Operator8/1 -> Logical Operator12/1, Logical Operator14/1
  Logical Operator9/1 -> Logical Operator15/2, Logical Operator12/2
  Logical Operator15/1 -> Logical Operator13/2, Logical Operator16/2
  Logical Operator14/1 -> Logical Operator11/1, Logical Operator13/1
  J-K Flip-Flop1/2 -> Logical Operator15/1
  NOT2/1 -> Logical Operator9/2
  J-K Flip-Flop2/2 -> Logical Operator16/1
  "EN "/1 -> NOT2/1, Logical Operator8/1
  Logical Operator11/1 -> Logical Operator10/1
  Logical Operator16/1 -> Logical Operator10/2
  Constant/1 -> Reset_Control1/2("JK ")
  Reset_Control1/1(J) -> J-K Flip-Flop/1
  Reset_Control1/2(K) -> J-K Flip-Flop/3
  Logical Operator12/1 -> Reset_Control3/2("JK ")
  Reset_Control3/1(J) -> J-K Flip-Flop1/1
  Reset_Control3/2(K) -> J-K Flip-Flop1/3
  Logical Operator13/1 -> Reset_Control4/2("JK ")
  Reset_Control4/1(J) -> J-K Flip-Flop2/1
  Reset_Control4/2(K) -> J-K Flip-Flop2/3
  Logical Operator10/1 -> Reset_Control2/2("JK ")
  Reset_Control2/1(J) -> J-K Flip-Flop3/1
  Reset_Control2/2(K) -> J-K Flip-Flop3/3
  J-K Flip-Flop3/2 -> Reset_Control1/3(A'), Reset_Control3/3(A'), Reset_Control4/3(A')
  EN_reset/1 -> Reset_Control1/1(EN_reset), Reset_Control3/1(EN_reset), Reset_Control4/1(EN_reset), Reset_Control2/1(EN_reset)

== system PONG/Next State /MOVE_YBall_CONTROLLED ( EN=0 >Up ;  EN=1 > Down ) 3 ==
  CLK : Inport
  EN1 : Inport  Port=2
  EN0 : Inport  Port=3
  EN_reset : Inport  Port=4
  Constant4 : Constant  OutDataTypeStr=boolean
  J-K Flip-Flop : simulink_extras/Flip Flops/J-K Flip-Flop  initial_condition=0
      settings: SourceProductName=Simulink
  J-K Flip-Flop1 : simulink_extras/Flip Flops/J-K Flip-Flop  initial_condition=1
      settings: SourceProductName=Simulink
  J-K Flip-Flop2 : simulink_extras/Flip Flops/J-K Flip-Flop  initial_condition=1
      settings: SourceProductName=Simulink
  Logical Operator12 : Logic  Operator=OR  IconShape=distinctive  AllPortsSameDT=off  OutDataTypeStr=boolean
  Logical Operator13 : Logic  Operator=OR  IconShape=distinctive  AllPortsSameDT=off  OutDataTypeStr=boolean
  Logical Operator{4,8..9,14..15} (5 alike) : Logic  IconShape=distinctive  AllPortsSameDT=off  OutDataTypeStr=boolean
  NOT1 : Logic  Operator=NOT  IconShape=distinctive  AllPortsSameDT=off  OutDataTypeStr=boolean
  Reset_Control : Subsystem  TreatAsAtomicUnit=on
  Reset_Control1 : Subsystem  TreatAsAtomicUnit=on
  Reset_Control2 : Subsystem  TreatAsAtomicUnit=on
  Scope : Scope  NumInputPorts=4
  E : Outport
  F : Outport  Port=2
  G : Outport  Port=3
  wires:
  CLK/1 -> Logical Operator4/2
  Logical Operator14/1 -> Logical Operator13/1
  Logical Operator9/1 -> Logical Operator12/2, Logical Operator15/2
  NOT1/1 -> Logical Operator9/2
  J-K Flip-Flop2/1 -> E/1, Scope/1
  Logical Operator8/1 -> Logical Operator14/1, Logical Operator12/1
  J-K Flip-Flop/2 -> Logical Operator9/1
  J-K Flip-Flop1/2 -> Logical Operator15/1
  Logical Operator15/1 -> Logical Operator13/2
  Logical Operator4/1 -> J-K Flip-Flop2/2, J-K Flip-Flop1/2, J-K Flip-Flop/2
  J-K Flip-Flop/1 -> Scope/3, G/1, Logical Operator8/2
  EN0/1 -> Logical Operator8/1, NOT1/1
  Logical Operator12/1 -> Reset_Control/2("JK ")
  Reset_Control/1(J) -> J-K Flip-Flop1/1
  Reset_Control/2(K) -> J-K Flip-Flop1/3
  Constant4/1 -> Reset_Control1/2("JK ")
  Reset_Control1/1(J) -> J-K Flip-Flop/1
  Reset_Control1/2(K) -> J-K Flip-Flop/3
  EN_reset/1 -> Reset_Control2/1(EN_reset), Reset_Control/1(EN_reset), Reset_Control1/1(EN_reset)
  Logical Operator13/1 -> Reset_Control2/2("JK ")
  Reset_Control2/1(J) -> J-K Flip-Flop2/1
  Reset_Control2/2(K) -> J-K Flip-Flop2/3
  J-K Flip-Flop2/2 -> Reset_Control1/3(E'), Reset_Control/3(E')
  J-K Flip-Flop1/1 -> Scope/2, F/1, Logical Operator14/2
  EN1/1 -> Logical Operator4/1

== system PONG/Paddle Control/Paddle Control0 ==
  PA : Inport
  PB : Inport  Port=2
  PC : Inport  Port=3
  PA1 : Inport  Port=4
  PB1 : Inport  Port=5
  PC1 : Inport  Port=6
  PA2 : Inport  Port=7
  PB2 : Inport  Port=8
  PC2 : Inport  Port=9
  E : Inport  Port=10
  F : Inport  Port=11
  G : Inport  Port=12
  Logical Operator : Logic  Operator=OR  Inputs=3  IconShape=distinctive  AllPortsSameDT=off  OutDataTypeStr=boolean
  Paddle Control0 : Subsystem  TreatAsAtomicUnit=on
  Paddle Control1 : Subsystem  TreatAsAtomicUnit=on
  Paddle Control2 : Subsystem  TreatAsAtomicUnit=on
  Paddle Check : Outport
  wires:
  Paddle Control0/1(Out1) -> Logical Operator/1
  Logical Operator/1 -> Paddle Check/1
  Paddle Control1/1(Out1) -> Logical Operator/2
  Paddle Control2/1(Out1) -> Logical Operator/3
  PA/1 -> Paddle Control0/4(PA)
  PB/1 -> Paddle Control0/5(PB)
  PC/1 -> Paddle Control0/6(PC)
  PA1/1 -> Paddle Control1/4(PA)
  PB1/1 -> Paddle Control1/5(PB)
  PC1/1 -> Paddle Control1/6(PC)
  PB2/1 -> Paddle Control2/5(PB)
  PA2/1 -> Paddle Control2/4(PA)
  PC2/1 -> Paddle Control2/6(PC)
  E/1 -> Paddle Control2/1(E), Paddle Control1/1(E), Paddle Control0/1(E)
  F/1 -> Paddle Control2/2(F), Paddle Control1/2(F), Paddle Control0/2(F)
  G/1 -> Paddle Control2/3(G), Paddle Control1/3(G), Paddle Control0/3(G)

== system PONG/Paddle Control/Paddle Control1 ==
  PA : Inport
  PB : Inport  Port=2
  PC : Inport  Port=3
  PA1 : Inport  Port=4
  PB1 : Inport  Port=5
  PC1 : Inport  Port=6
  PA2 : Inport  Port=7
  PB2 : Inport  Port=8
  PC2 : Inport  Port=9
  E : Inport  Port=10
  F : Inport  Port=11
  G : Inport  Port=12
  Logical Operator : Logic  Operator=OR  Inputs=3  IconShape=distinctive  AllPortsSameDT=off  OutDataTypeStr=boolean
  Paddle Control0 : Subsystem  TreatAsAtomicUnit=on
  Paddle Control1 : Subsystem  TreatAsAtomicUnit=on
  Paddle Control2 : Subsystem  TreatAsAtomicUnit=on
  Paddle Check : Outport
  wires:
  G/1 -> Paddle Control0/3(G), Paddle Control1/3(G), Paddle Control2/3(G)
  F/1 -> Paddle Control0/2(F), Paddle Control1/2(F), Paddle Control2/2(F)
  E/1 -> Paddle Control0/1(E), Paddle Control1/1(E), Paddle Control2/1(E)
  PC2/1 -> Paddle Control2/6(PC)
  PA2/1 -> Paddle Control2/4(PA)
  PB2/1 -> Paddle Control2/5(PB)
  PC1/1 -> Paddle Control1/6(PC)
  PB1/1 -> Paddle Control1/5(PB)
  PA1/1 -> Paddle Control1/4(PA)
  PC/1 -> Paddle Control0/6(PC)
  PB/1 -> Paddle Control0/5(PB)
  PA/1 -> Paddle Control0/4(PA)
  Paddle Control2/1(Out1) -> Logical Operator/3
  Paddle Control1/1(Out1) -> Logical Operator/2
  Logical Operator/1 -> Paddle Check/1
  Paddle Control0/1(Out1) -> Logical Operator/1

== system PONG/Paddle Control/Position Control ==
  A : Inport
  B : Inport  Port=2
  C : Inport  Port=3
  D : Inport  Port=4
  Logical Operator : Logic  Inputs=4  IconShape=distinctive  AllPortsSameDT=off  OutDataTypeStr=boolean
  NXOR : Logic  Operator=NXOR  IconShape=distinctive  AllPortsSameDT=off  OutDataTypeStr=boolean
  NXOR1 : Logic  Operator=NXOR  IconShape=distinctive  AllPortsSameDT=off  OutDataTypeStr=boolean
  XOR1 : Logic  Operator=XOR  IconShape=distinctive  AllPortsSameDT=off  OutDataTypeStr=boolean
  Position Check : Outport
  wires:
  Logical Operator/1 -> Position Check/1
  C/1 -> XOR1/2, Logical Operator/4, NXOR1/1
  D/1 -> NXOR1/2
  A/1 -> NXOR/1
  B/1 -> XOR1/1, NXOR/2
  NXOR1/1 -> Logical Operator/3
  XOR1/1 -> Logical Operator/2
  NXOR/1 -> Logical Operator/1

== system PONG/Paddle Control/Position Control1 ==
  A : Inport
  B : Inport  Port=2
  C : Inport  Port=3
  D : Inport  Port=4
  Logical Operator : Logic  Inputs=4  IconShape=distinctive  AllPortsSameDT=off  OutDataTypeStr=boolean
  NXOR : Logic  Operator=NXOR  IconShape=distinctive  AllPortsSameDT=off  OutDataTypeStr=boolean
  NXOR1 : Logic  Operator=NXOR  IconShape=distinctive  AllPortsSameDT=off  OutDataTypeStr=boolean
  XOR1 : Logic  Operator=XOR  IconShape=distinctive  AllPortsSameDT=off  OutDataTypeStr=boolean
  Position Check : Outport
  wires:
  NXOR/1 -> Logical Operator/1
  XOR1/1 -> Logical Operator/3
  NXOR1/1 -> Logical Operator/4
  B/1 -> Logical Operator/2, NXOR/2, XOR1/1
  A/1 -> NXOR/1
  D/1 -> NXOR1/2
  C/1 -> XOR1/2, NXOR1/1
  Logical Operator/1 -> Position Check/1

== system PONG/Paddle DEMUXER0/1PaddleDEMUXER0 ==
  PA : Inport
  PB : Inport  Port=2
  PC : Inport  Port=3
  Logical Operator{,1..7} (8 alike) : Logic  Inputs=3  IconShape=distinctive  AllPortsSameDT=off  OutDataTypeStr=boolean
  NOT : Logic  Operator=NOT  IconShape=distinctive  AllPortsSameDT=off  OutDataTypeStr=boolean
  NOT1 : Logic  Operator=NOT  IconShape=distinctive  AllPortsSameDT=off  OutDataTypeStr=boolean
  NOT2 : Logic  Operator=NOT  IconShape=distinctive  AllPortsSameDT=off  OutDataTypeStr=boolean
  Out1 : Outport
  Out2 : Outport  Port=2
  Out3 : Outport  Port=3
  Out4 : Outport  Port=4
  Out5 : Outport  Port=5
  Out6 : Outport  Port=6
  Out7 : Outport  Port=7
  Out8 : Outport  Port=8
  wires:
  Logical Operator/1 -> Out1/1
  Logical Operator1/1 -> Out2/1
  Logical Operator3/1 -> Out4/1
  Logical Operator2/1 -> Out3/1
  Logical Operator7/1 -> Out8/1
  Logical Operator6/1 -> Out7/1
  Logical Operator5/1 -> Out6/1
  Logical Operator4/1 -> Out5/1
  PC/1 -> Logical Operator6/1, Logical Operator7/3, Logical Operator5/1, Logical Operator4/1, NOT2/1
  NOT/1 -> Logical Operator/3, Logical Operator2/3, Logical Operator6/3, Logical Operator4/3
  NOT1/1 -> Logical Operator5/2, Logical Operator4/2, Logical Operator1/2, Logical Operator/2
  NOT2/1 -> Logical Operator/1, Logical Operator3/1, Logical Operator2/1, Logical Operator1/1
  PA/1 -> Logical Operator7/1, Logical Operator5/3, Logical Operator3/3, Logical Operator1/3, NOT/1
  PB/1 -> Logical Operator2/2, Logical Operator6/2, Logical Operator7/2, Logical Operator3/2, NOT1/1

== system PONG/Paddle DEMUXER0/1PaddleDEMUXER2 ==
  PA : Inport
  PB : Inport  Port=2
  PC : Inport  Port=3
  Logical Operator{,1..7} (8 alike) : Logic  Inputs=3  IconShape=distinctive  AllPortsSameDT=off  OutDataTypeStr=boolean
  NOT : Logic  Operator=NOT  IconShape=distinctive  AllPortsSameDT=off  OutDataTypeStr=boolean
  NOT1 : Logic  Operator=NOT  IconShape=distinctive  AllPortsSameDT=off  OutDataTypeStr=boolean
  NOT2 : Logic  Operator=NOT  IconShape=distinctive  AllPortsSameDT=off  OutDataTypeStr=boolean
  Out1 : Outport
  Out2 : Outport  Port=2
  Out3 : Outport  Port=3
  Out4 : Outport  Port=4
  Out5 : Outport  Port=5
  Out6 : Outport  Port=6
  Out7 : Outport  Port=7
  Out8 : Outport  Port=8
  wires:
  Logical Operator/1 -> Out1/1
  Logical Operator1/1 -> Out2/1
  Logical Operator3/1 -> Out4/1
  Logical Operator2/1 -> Out3/1
  Logical Operator7/1 -> Out8/1
  Logical Operator6/1 -> Out7/1
  Logical Operator5/1 -> Out6/1
  Logical Operator4/1 -> Out5/1
  PA/1 -> Logical Operator6/1, Logical Operator7/3, Logical Operator5/1, Logical Operator4/1, NOT2/1
  NOT/1 -> Logical Operator/3, Logical Operator2/3, Logical Operator6/3, Logical Operator4/3
  NOT1/1 -> Logical Operator5/2, Logical Operator4/2, Logical Operator1/2, Logical Operator/2
  NOT2/1 -> Logical Operator/1, Logical Operator3/1, Logical Operator2/1, Logical Operator1/1
  PC/1 -> Logical Operator7/1, Logical Operator5/3, Logical Operator3/3, Logical Operator1/3, NOT/1
  PB/1 -> Logical Operator2/2, Logical Operator6/2, Logical Operator7/2, Logical Operator3/2, NOT1/1

== system PONG/Paddle DEMUXER0/2PaddleDEMUXER1 ==
  PA : Inport
  PB : Inport  Port=2
  PC : Inport  Port=3
  Logical Operator{,1..7} (8 alike) : Logic  Inputs=3  IconShape=distinctive  AllPortsSameDT=off  OutDataTypeStr=boolean
  NOT : Logic  Operator=NOT  IconShape=distinctive  AllPortsSameDT=off  OutDataTypeStr=boolean
  NOT1 : Logic  Operator=NOT  IconShape=distinctive  AllPortsSameDT=off  OutDataTypeStr=boolean
  NOT2 : Logic  Operator=NOT  IconShape=distinctive  AllPortsSameDT=off  OutDataTypeStr=boolean
  Out1 : Outport
  Out2 : Outport  Port=2
  Out3 : Outport  Port=3
  Out4 : Outport  Port=4
  Out5 : Outport  Port=5
  Out6 : Outport  Port=6
  Out7 : Outport  Port=7
  Out8 : Outport  Port=8
  wires:
  PB/1 -> NOT1/1, Logical Operator3/2, Logical Operator7/2, Logical Operator6/2, Logical Operator2/2
  PC/1 -> NOT/1, Logical Operator1/3, Logical Operator3/3, Logical Operator5/3, Logical Operator7/1
  NOT2/1 -> Logical Operator1/1, Logical Operator2/1, Logical Operator3/1, Logical Operator/1
  NOT1/1 -> Logical Operator/2, Logical Operator1/2, Logical Operator4/2, Logical Operator5/2
  NOT/1 -> Logical Operator4/3, Logical Operator6/3, Logical Operator2/3, Logical Operator/3
  PA/1 -> NOT2/1, Logical Operator4/1, Logical Operator5/1, Logical Operator7/3, Logical Operator6/1
  Logical Operator4/1 -> Out5/1
  Logical Operator5/1 -> Out6/1
  Logical Operator6/1 -> Out7/1
  Logical Operator7/1 -> Out8/1
  Logical Operator2/1 -> Out3/1
  Logical Operator3/1 -> Out4/1
  Logical Operator1/1 -> Out2/1
  Logical Operator/1 -> Out1/1

== system PONG/Paddle DEMUXER1/1PaddleDEMUXER0 ==
  PA : Inport
  PB : Inport  Port=2
  PC : Inport  Port=3
  Logical Operator{,1..7} (8 alike) : Logic  Inputs=3  IconShape=distinctive  AllPortsSameDT=off  OutDataTypeStr=boolean
  NOT : Logic  Operator=NOT  IconShape=distinctive  AllPortsSameDT=off  OutDataTypeStr=boolean
  NOT1 : Logic  Operator=NOT  IconShape=distinctive  AllPortsSameDT=off  OutDataTypeStr=boolean
  NOT2 : Logic  Operator=NOT  IconShape=distinctive  AllPortsSameDT=off  OutDataTypeStr=boolean
  Out1 : Outport
  Out2 : Outport  Port=2
  Out3 : Outport  Port=3
  Out4 : Outport  Port=4
  Out5 : Outport  Port=5
  Out6 : Outport  Port=6
  Out7 : Outport  Port=7
  Out8 : Outport  Port=8
  wires:
  PB/1 -> NOT1/1, Logical Operator3/2, Logical Operator7/2, Logical Operator6/2, Logical Operator2/2
  PC/1 -> NOT/1, Logical Operator1/3, Logical Operator3/3, Logical Operator5/3, Logical Operator7/1
  NOT2/1 -> Logical Operator1/1, Logical Operator2/1, Logical Operator3/1, Logical Operator/1
  NOT1/1 -> Logical Operator/2, Logical Operator1/2, Logical Operator4/2, Logical Operator5/2
  NOT/1 -> Logical Operator4/3, Logical Operator6/3, Logical Operator2/3, Logical Operator/3
  PA/1 -> NOT2/1, Logical Operator4/1, Logical Operator5/1, Logical Operator7/3, Logical Operator6/1
  Logical Operator4/1 -> Out5/1
  Logical Operator5/1 -> Out6/1
  Logical Operator6/1 -> Out7/1
  Logical Operator7/1 -> Out8/1
  Logical Operator2/1 -> Out3/1
  Logical Operator3/1 -> Out4/1
  Logical Operator1/1 -> Out2/1
  Logical Operator/1 -> Out1/1

== system PONG/Paddle DEMUXER1/1PaddleDEMUXER1 ==
  PA : Inport
  PB : Inport  Port=2
  PC : Inport  Port=3
  Logical Operator{,1..7} (8 alike) : Logic  Inputs=3  IconShape=distinctive  AllPortsSameDT=off  OutDataTypeStr=boolean
  NOT : Logic  Operator=NOT  IconShape=distinctive  AllPortsSameDT=off  OutDataTypeStr=boolean
  NOT1 : Logic  Operator=NOT  IconShape=distinctive  AllPortsSameDT=off  OutDataTypeStr=boolean
  NOT2 : Logic  Operator=NOT  IconShape=distinctive  AllPortsSameDT=off  OutDataTypeStr=boolean
  Out1 : Outport
  Out2 : Outport  Port=2
  Out3 : Outport  Port=3
  Out4 : Outport  Port=4
  Out5 : Outport  Port=5
  Out6 : Outport  Port=6
  Out7 : Outport  Port=7
  Out8 : Outport  Port=8
  wires:
  Logical Operator/1 -> Out1/1
  Logical Operator1/1 -> Out2/1
  Logical Operator3/1 -> Out4/1
  Logical Operator2/1 -> Out3/1
  Logical Operator7/1 -> Out8/1
  Logical Operator6/1 -> Out7/1
  Logical Operator5/1 -> Out6/1
  Logical Operator4/1 -> Out5/1
  PA/1 -> Logical Operator6/1, Logical Operator7/3, Logical Operator5/1, Logical Operator4/1, NOT2/1
  NOT/1 -> Logical Operator/3, Logical Operator2/3, Logical Operator6/3, Logical Operator4/3
  NOT1/1 -> Logical Operator5/2, Logical Operator4/2, Logical Operator1/2, Logical Operator/2
  NOT2/1 -> Logical Operator/1, Logical Operator3/1, Logical Operator2/1, Logical Operator1/1
  PC/1 -> Logical Operator7/1, Logical Operator5/3, Logical Operator3/3, Logical Operator1/3, NOT/1
  PB/1 -> Logical Operator2/2, Logical Operator6/2, Logical Operator7/2, Logical Operator3/2, NOT1/1
